simulink model "Quadcopter_LQR_6DOF"  (R2022a)
settings: Solver=VariableStepAuto  StartTime=0.0  StopTime=60  RelTol=1e-3
undefined symbols (not defined in the file): A, B, C, Klqr
settings Model: Creator=creec  LastModifiedBy=creec

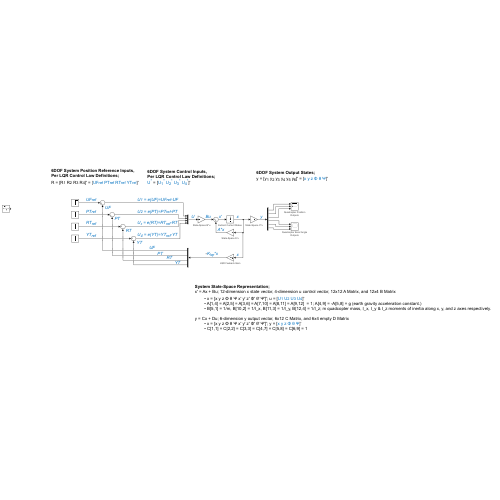
[thumbnail: Simulink's stored preview of the top-level diagram]
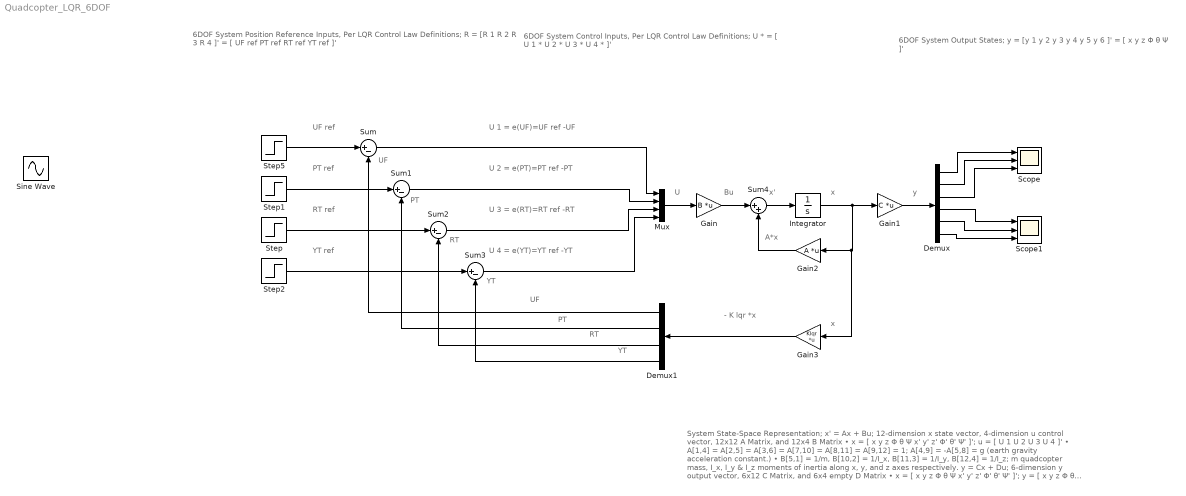
== system Quadcopter_LQR_6DOF ==
  note: RT
  note: PT
  note: 6DOF System Control Inputs,
      | Per LQR Control Law Definitions;
      | U * = [ U 1 * U 2 * U 3 * U 4 * ]'
  note: 6DOF System Position Reference Inputs,
      | Per LQR Control Law Definitions;
      | R = [R 1 R 2 R 3 R 4 ]' = [ UF ref PT ref RT ref YT ref ]'
  note: PT ref
  note: RT ref
  note: U 1 = e(UF)=UF ref -UF
  note: UF ref
  note: YT ref
  note: UF
  note: YT
  note: U 2 = e(PT)=PT ref -PT
  note: U 3 = e(RT)=RT ref -RT
  note: U 4 = e(YT)=YT ref -YT
  note: UF
  note: PT
  note: RT
  note: YT
  note: U
  note: Bu
  note: x'
  note: x
  note: y
  note: A*x
  note: x
  note: - K lqr *x
  note: System State-Space Representation;
      | x' = Ax + Bu; 12-dimension x state vector, 4-dimension u control vector, 12x12 A Matrix, and 12x4 B Matrix
      | • x = [ x y z Φ θ Ψ x' y' z' Φ' θ' Ψ' ]'; u = [ U 1 U 2 U 3 U 4 ]'
      | • A[1,4] = A[2,5] = A[3,6] = A[7,10] = A[8,11] = A[9,12] = 1; A[4,9] = -A[5,8] = g (earth gravity acceleration constant.)
      | • B[5,1] = 1/m, B[10,2] = 1/I_x, B[11,3] = 1/I_y, B[12,4] = 1/I_z; m quadcopter mass, I_x, I_y & I_z moments of inertia along x, y, and z axes respectively.
      |
      | y = Cx + Du; 6-dimension y output vector, 6x12 C Matrix, and 6x4 empty D Matrix
      | • x = [ x y z Φ θ Ψ x' y' z' Φ' θ' Ψ' ]'; y = [ x y z Φ θ Ψ ]'
      | • C[1,1] = C[2,2] = C[3,3] = C[4,7] = C[5,8] = C[6,9] = 1
  note: 6DOF System Output States;
      | y = [y 1 y 2 y 3 y 4 y 5 y 6 ]' = [ x y z Φ θ Ψ ]'
  Demux : Demux  Outputs=6
  Demux1 : Demux
  Gain : Gain  Gain=B  Multiplication=Matrix(K*u)
      settings: AttributesFormatString=State-Space B*u
  Gain1 : Gain  Gain=C  Multiplication=Matrix(K*u)
      settings: AttributesFormatString=State-Space C*x
  Gain2 : Gain  Gain=A  Multiplication=Matrix(K*u)
      settings: AttributesFormatString=State-Space A*x
  Gain3 : Gain  Gain=Klqr  Multiplication=Matrix(K*u)
      settings: AttributesFormatString=LQR Feeback Gain
  Integrator : Integrator
      settings: AttributesFormatString=Extract Current States
  Mux : Mux
  Scope : Scope  NumInputPorts=3
      settings: AttributesFormatString=|
      | Quadcopter Position
      | Outputs
  Scope1 : Scope  NumInputPorts=3
      settings: AttributesFormatString=|
      | Quadcopter Euler Angle
      | Outputs
  Sine Wave : Sin  Frequency=90/2*pi  SampleTime=0
  Step : Step  Time=30  After=1.5  SampleTime=0
  Step1 : Step  Time=10  After=-2  SampleTime=0
  Step2 : Step  Time=30  After=1.5  SampleTime=0
  Step5 : Step  SampleTime=0
  Sum{,1..3} (4 alike) : Sum  Inputs=|+-
  Sum4 : Sum  Inputs=|++
  wires:
  Demux/3 -> Scope/3
  Integrator/1 -> Gain1/1, Gain3/1, Gain2/1
  Demux/2 -> Scope/2
  Demux/1 -> Scope/1
  Gain2/1 -> Sum4/2
  Mux/1 -> Gain/1
  Step/1 -> Sum2/1
  Step5/1 -> Sum/1
  Step2/1 -> Sum3/1
  Sum4/1 -> Integrator/1
  Demux/6 -> Scope1/3
  Demux/4 -> Scope1/1
  Gain1/1 -> Demux/1
  Gain/1 -> Sum4/1
  Demux/5 -> Scope1/2
  Step1/1 -> Sum1/1
  Gain3/1 -> Demux1/1
  Demux1/1 -> Sum/2
  Demux1/2 -> Sum1/2
  Demux1/3 -> Sum2/2
  Demux1/4 -> Sum3/2
  Sum/1 -> Mux/1
  Sum1/1 -> Mux/2
  Sum2/1 -> Mux/3
  Sum3/1 -> Mux/4
